simulink subsystem "stack_subsystem_model"  (R2023a)
settings: Solver=VariableStepAuto  StartTime=0.0  StopTime=10.0  RelTol=1e-3
undefined symbols (not defined in the file): constants, coolant_initial_temperature, coolant_num_layers, coolant_num_passes, coolant_w_channels, dewpoint_temperature_degC, env_p, h2_molar_concentration, hydrogen, inlet_flow_lpmin, inlet_pressure_barg, inlet_temperature_degC, oxygen, stack_area, stack_num_cells, stoichiometry
libraries: fl_lib x39, nesl_utility x31
(part 1 of 2)
settings Model: Creator=stefan.notter  LastModifiedBy=adrian.taveras
settings OptimizationCC: ReuseModelBlockBuffer=off

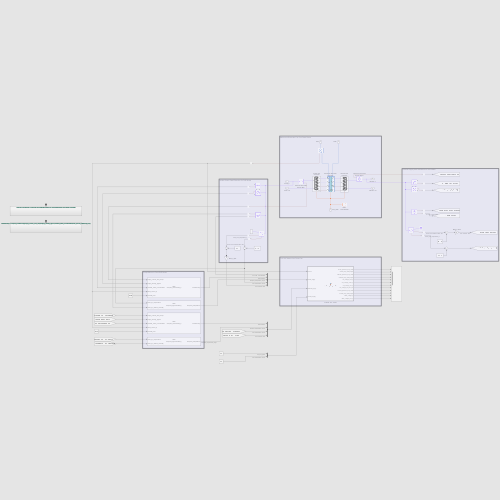
[thumbnail: Simulink's stored preview of the top-level diagram]
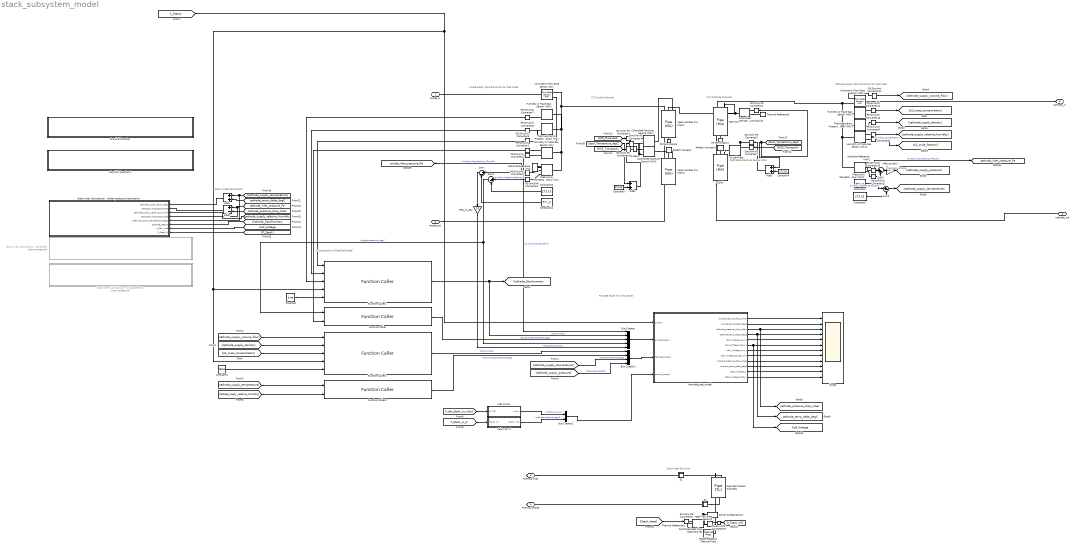
== system stack_subsystem_model ==
  note: Stack-model-Parameters
  note: Computations to Feed DoE Model
  note: Anode Supply Data Extraction for DoE Model
  note: P10 DoE Model from PowerCell
  note: Cathode Supply Data Extraction for DoE Model
  note: FCS Cathode Channels
  note: FCS Anode Channels
  note: Stack Heat Emission
  Absolute Reference (MA) : fl_lib/Moist Air/Elements/Absolute Reference (MA)
  Absolute Reference (MA)1 : fl_lib/Moist Air/Elements/Absolute Reference (MA)
  Add1 : Sum
  Add2 : Sum  Inputs=+-
  Add3 : Sum
  Add4 : Sum
  Bus Creator : BusCreator  Inputs=h2_molar_concentration,stoichiometry,dewpoint_temperature_degC,inlet_temperature_degC,inlet_pressure_barg  OutDataTypeStr=Bus: anode_supply
  Bus Creator1 : BusCreator  Inputs=stoichiometry,dewpoint_temperature_degC,inlet_temperature_degC,inlet_pressure_barg  OutDataTypeStr=Bus: cathode_supply
  Bus Creator2 : BusCreator  Inputs=inlet_flow_lpmin,inlet_temperature_degC  OutDataTypeStr=Bus: coolant_supply
  Cond. : fl_lib/Moist Air/Elements/Pipe (MA)  length=1 m  area=1 m^2  Dh=.1 m  length_add=.1 m  roughness=15e-6 m  Re_lam=2000  Re_tur=4000  shape_factor=64  Nu_lam=3.66  wall_condensation=simscape.enum.onoff.off  RH_ws=1  time_constant=1e-3 s  moisture_trace_gas_source=foundation.enum.moisture_trace_gas_source.controlled  moisture_source_spec=foundation.enum.moisture_source_spec.vapor  moisture_mass_flow=0 kg/s  moisture_temperature_spec=foundation.enum.temperature_spec.atmospheric  moisture_temperature=293.15 K  trace_gas_mass_flow=0 kg/s  trace_gas_temperature_spec=foundation.enum.temperature_spec.atmospheric  trace_gas_temperature=293.15 K  p_I_specify=off  p_I_priority=High  p_I=0.101325 MPa  p_I_nominal_specify=off  p_I_nominal_unit=MPa  p_I_nominal_value=1  T_I_specify=off  T_I_priority=High  T_I=293.15 K  T_I_nominal_specify=off  T_I_nominal_unit=K  T_I_nominal_value=1  RH_I_specify=off  RH_I_priority=High  RH_I=0  RH_I_nominal_specify=off  RH_I_nominal_unit=1  RH_I_nominal_value=1  x_w_I_specify=off  x_w_I_priority=None  x_w_I=0  x_w_I_nominal_specify=off  x_w_I_nominal_unit=1  x_w_I_nominal_value=1  y_w_I_specify=off  y_w_I_priority=None  y_w_I=0  y_w_I_nominal_specify=off  y_w_I_nominal_unit=1  y_w_I_nominal_value=1  HR_I_specify=off  HR_I_priority=None  HR_I=0  HR_I_nominal_specify=off  HR_I_nominal_unit=1  HR_I_nominal_value=1  x_g_I_specify=off  x_g_I_priority=High  x_g_I=0  x_g_I_nominal_specify=off  x_g_I_nominal_unit=1  x_g_I_nominal_value=1  y_g_I_specify=off  y_g_I_priority=None  y_g_I=0  y_g_I_nominal_specify=off  y_g_I_nominal_unit=1  y_g_I_nominal_value=1
      settings: InternalSimscapePortConfiguration="{\"Bottom\":[],\"Left\":[{\"id\":\"A\",\"label\":\"A\",\"type\":\"foundation.moist_air.moist_air\"},{\"id\":\"H\",\"label\":\"H\",\"type\":\"foundation.thermal.thermal\"},{\"id\":\"S\",\"label\":\"S\",\"type\":\"foundation.moist_air.moist_air_source\"}],\"Right\":[{\"id\":\"B\",\"label\":\"B\",\"type\":\"foundation.moist_air.moist_air\"},{\"id\":\"W\",\"label\":\"W\",\"type\":\"output\"},{\"id\":\"F\",\"label\":\"F\",\"type\":\"output\"}],\"Top\":[]}"
  Constant : Constant  Value=true  OutDataTypeStr=boolean
  Constant1 : Constant  Value=false  OutDataTypeStr=boolean
  Constant11 : Constant  Value=env_p
  Constant12 : Constant  Value=273.15
  Constant2 : Constant  Value=env_p
  Constant3 : Constant  Value=273.15
  Constant4 : Constant  Value=273.16
  Constant5 : Constant  Value=273.16
  Controlled Temperature Source : fl_lib/Thermal/Thermal Sources/Controlled Temperature Source
  Controlled Heat Flow Rate Source1 : fl_lib/Thermal/Thermal Sources/Controlled Heat Flow Rate Source
  Controlled Moisture Source (MA)1 : fl_lib/Moist Air/Sources/Moisture & Trace Gas Sources/Controlled Moisture Source (MA)  moisture_source_spec=foundation.enum.moisture_source_spec.vapor  Phi_S_specify=off  Phi_S_priority=None  Phi_S=0 kW  Phi_S_nominal_specify=off  Phi_S_nominal_unit=kW  Phi_S_nominal_value=1  mdot_w_S_specify=off  mdot_w_S_priority=None  mdot_w_S=0 kg/s  mdot_w_S_nominal_specify=off  mdot_w_S_nominal_unit=kg/s  mdot_w_S_nominal_value=1
      settings: InternalSimscapePortConfiguration="{\"Bottom\":[],\"Left\":[{\"id\":\"S\",\"label\":\"S\",\"type\":\"foundation.moist_air.moist_air_source\"}],\"Right\":[{\"id\":\"M\",\"label\":\"M\",\"type\":\"input\"},{\"id\":\"T\",\"label\":\"T\",\"type\":\"input\"}],\"Top\":[]}"
  Controlled Moisture Source (MA)2 : fl_lib/Moist Air/Sources/Moisture & Trace Gas Sources/Controlled Moisture Source (MA)  moisture_source_spec=foundation.enum.moisture_source_spec.vapor  Phi_S_specify=off  Phi_S_priority=None  Phi_S=0 kW  Phi_S_nominal_specify=off  Phi_S_nominal_unit=kW  Phi_S_nominal_value=1  mdot_w_S_specify=off  mdot_w_S_priority=None  mdot_w_S=0 kg/s  mdot_w_S_nominal_specify=off  mdot_w_S_nominal_unit=kg/s  mdot_w_S_nominal_value=1
      settings: InternalSimscapePortConfiguration="{\"Bottom\":[],\"Left\":[{\"id\":\"S\",\"label\":\"S\",\"type\":\"foundation.moist_air.moist_air_source\"}],\"Right\":[{\"id\":\"M\",\"label\":\"M\",\"type\":\"input\"},{\"id\":\"T\",\"label\":\"T\",\"type\":\"input\"}],\"Top\":[]}"
  Fuel Cell Coolant Channels : fl_lib/Thermal Liquid/Elements/Pipe (TL)  length=sqrt(stack_area) * coolant_num_passes cm  area=coolant_w_channels^2 * coolant_num_layers cm^2  Dh=coolant_w_channels cm  length_add=10 cm  roughness=15e-5 m  Re_lam=2000  Re_tur=4000  shape_factor=64  Nu_lam=3.66  dynamic_compressibility=simscape.enum.onoff.on  inertia=simscape.enum.onoff.off  p0=coolant_initial_pressure MPa  T0=coolant_initial_temperature K  mdot0=0 kg/s
  Function Caller : FunctionCaller  FunctionPrototype=dewpoint_temperature = dewpoint_approximation(moist_air_temperature,moist_air_relative_humidity)  InputArgumentSpecifications=<Enter example>  OutputArgumentSpecifications=<Enter example>
  Function Caller1 : FunctionCaller  FunctionPrototype=stoichiometry = compute_stoichiometry(supply_volume_flow_m3ps,supply_density_kgpm3,reactant_mass_concentration,stack_current_A,isanode_bool)  InputArgumentSpecifications=<Enter example>  OutputArgumentSpecifications=<Enter example>
  Function Caller2 : FunctionCaller  FunctionPrototype=stoichiometry = compute_stoichiometry(supply_volume_flow_m3ps,supply_density_kgpm3,reactant_mass_concentration,stack_current_A,isanode_bool)  InputArgumentSpecifications=<Enter example>  OutputArgumentSpecifications=<Enter example>
  Function Caller3 : FunctionCaller  FunctionPrototype=dewpoint_temperature = dewpoint_approximation(moist_air_temperature,moist_air_relative_humidity)  InputArgumentSpecifications=<Enter example>  OutputArgumentSpecifications=<Enter example>
  Heat Flow Rate Sensor1 : fl_lib/Thermal/Thermal Sensors/Heat Flow Rate Sensor
  Humidity & Trace Gas Sensor (MA) : fl_lib/Moist Air/Sensors/Humidity & Trace Gas Sensor (MA)  moisture_on=true  moisture_spec=foundation.enum.moisture_spec.relative_humidity  trace_gas_on=true  trace_gas_spec=foundation.enum.trace_gas_spec.mole_fraction
      settings: InternalSimscapePortConfiguration="{\"Bottom\":[],\"Left\":[{\"id\":\"A\",\"label\":\"A\",\"type\":\"foundation.moist_air.moist_air\"}],\"Right\":[{\"id\":\"W\",\"label\":\"W\",\"type\":\"output\"},{\"id\":\"G\",\"label\":\"G\",\"type\":\"output\"}],\"Top\":[]}"
  Humidity & Trace Gas Sensor (MA)1 : fl_lib/Moist Air/Sensors/Humidity & Trace Gas Sensor (MA)  moisture_on=true  moisture_spec=foundation.enum.moisture_spec.relative_humidity  trace_gas_on=true  trace_gas_spec=foundation.enum.trace_gas_spec.mass_fraction
      settings: InternalSimscapePortConfiguration="{\"Bottom\":[],\"Left\":[{\"id\":\"A\",\"label\":\"A\",\"type\":\"foundation.moist_air.moist_air\"}],\"Right\":[{\"id\":\"W\",\"label\":\"W\",\"type\":\"output\"},{\"id\":\"G\",\"label\":\"G\",\"type\":\"output\"}],\"Top\":[]}"
  Humidity & Trace Gas Sensor (MA)2 : fl_lib/Moist Air/Sensors/Humidity & Trace Gas Sensor (MA)  moisture_on=true  moisture_spec=foundation.enum.moisture_spec.relative_humidity  trace_gas_on=true  trace_gas_spec=foundation.enum.trace_gas_spec.mole_fraction
      settings: InternalSimscapePortConfiguration="{\"Bottom\":[],\"Left\":[{\"id\":\"A\",\"label\":\"A\",\"type\":\"foundation.moist_air.moist_air\"}],\"Right\":[{\"id\":\"W\",\"label\":\"W\",\"type\":\"output\"},{\"id\":\"G\",\"label\":\"G\",\"type\":\"output\"}],\"Top\":[]}"
  Humidity & Trace Gas Sensor (MA)3 : fl_lib/Moist Air/Sensors/Humidity & Trace Gas Sensor (MA)  moisture_on=true  moisture_spec=foundation.enum.moisture_spec.relative_humidity  trace_gas_on=true  trace_gas_spec=foundation.enum.trace_gas_spec.mass_fraction
      settings: InternalSimscapePortConfiguration="{\"Bottom\":[],\"Left\":[{\"id\":\"A\",\"label\":\"A\",\"type\":\"foundation.moist_air.moist_air\"}],\"Right\":[{\"id\":\"W\",\"label\":\"W\",\"type\":\"output\"},{\"id\":\"G\",\"label\":\"G\",\"type\":\"output\"}],\"Top\":[]}"
  Kelvin to °C : Subsystem
  M3s to lpm : Subsystem
  MPa_to_Bar : Gain  Gain=10
  MPa_to_Bar1 : Gain  Gain=10
  PS Gain2 : fl_lib/Physical Signals/Functions/PS Gain  gain=-1
  PS Terminator1 : fl_lib/Physical Signals/Sinks/PS Terminator
  PS Terminator6 : fl_lib/Physical Signals/Sinks/PS Terminator
  PS-Simulink Converter{1..2,4..9,11..14} (12 alike) : nesl_utility/PS-Simulink Converter  PhysicalDomain=network_engine_domain  SubClassName=ps_output  LeftPortType=input  RightPortType=output  PseudoPeriodic=off  Frequencies=[]  VectorFormat=inherit  Unit=inherit  AffineConversion=off
  PS-Simulink Converter10 : nesl_utility/PS-Simulink Converter  PhysicalDomain=network_engine_domain  SubClassName=ps_output  LeftPortType=input  RightPortType=output  PseudoPeriodic=off  Frequencies=[]  VectorFormat=inherit  Unit=MPa  AffineConversion=off
  PS-Simulink Converter16 : nesl_utility/PS-Simulink Converter  PhysicalDomain=network_engine_domain  SubClassName=ps_output  LeftPortType=input  RightPortType=output  PseudoPeriodic=off  Frequencies=[]  VectorFormat=1-D array  Unit=kW  AffineConversion=off
  PS-Simulink Converter3 : nesl_utility/PS-Simulink Converter  PhysicalDomain=network_engine_domain  SubClassName=ps_output  LeftPortType=input  RightPortType=output  PseudoPeriodic=off  Frequencies=[]  VectorFormat=inherit  Unit=MPa  AffineConversion=off
  PS100-P02Stack Thermal Mass : fl_lib/Thermal/Thermal Elements/Thermal Mass  mass_type=foundation.enum.constant_variable.constant  mass=stack_thermal_mass kg  sp_heat=stack_specific_heat J/kg/K  mass_min=1e-6 kg  num_ports=foundation.enum.numPorts2.one  m_specify=off  m_priority=High  m=1 kg  m_nominal_specify=off  m_nominal_unit=kg  m_nominal_value=1  T_specify=on  T_priority=High  T=coolant_initial_temperature K  T_nominal_specify=off  T_nominal_unit=K  T_nominal_value=1  Q_specify=off  Q_priority=None  Q=20e3 W  Q_nominal_specify=off  Q_nominal_unit=W  Q_nominal_value=1
  Perfect Insulator : fl_lib/Thermal/Thermal Elements/Perfect Insulator  T_specify=off  T_priority=None  T=293.15 K  T_nominal_specify=off  T_nominal_unit=K  T_nominal_value=1
  Perfect Insulator1 : fl_lib/Thermal/Thermal Elements/Perfect Insulator  T_specify=off  T_priority=None  T=293.15 K  T_nominal_specify=off  T_nominal_unit=K  T_nominal_value=1
  Pipe (MA) : fl_lib/Moist Air/Elements/Pipe (MA)  length=1 m  area=1 m^2  Dh=.1 m  length_add=.1 m  roughness=15e-6 m  Re_lam=2000  Re_tur=4000  shape_factor=64  Nu_lam=3.66  wall_condensation=simscape.enum.onoff.off  RH_ws=1  time_constant=1e-3 s  moisture_trace_gas_source=foundation.enum.moisture_trace_gas_source.none  moisture_source_spec=foundation.enum.moisture_source_spec.vapor  moisture_mass_flow=0 kg/s  moisture_temperature_spec=foundation.enum.temperature_spec.atmospheric  moisture_temperature=293.15 K  trace_gas_mass_flow=0 kg/s  trace_gas_temperature_spec=foundation.enum.temperature_spec.atmospheric  trace_gas_temperature=293.15 K  p_I_specify=off  p_I_priority=High  p_I=0.101325 MPa  p_I_nominal_specify=off  p_I_nominal_unit=MPa  p_I_nominal_value=1  T_I_specify=off  T_I_priority=High  T_I=293.15 K  T_I_nominal_specify=off  T_I_nominal_unit=K  T_I_nominal_value=1  RH_I_specify=off  RH_I_priority=High  RH_I=0  RH_I_nominal_specify=off  RH_I_nominal_unit=1  RH_I_nominal_value=1  x_w_I_specify=off  x_w_I_priority=None  x_w_I=0  x_w_I_nominal_specify=off  x_w_I_nominal_unit=1  x_w_I_nominal_value=1  y_w_I_specify=off  y_w_I_priority=None  y_w_I=0  y_w_I_nominal_specify=off  y_w_I_nominal_unit=1  y_w_I_nominal_value=1  HR_I_specify=off  HR_I_priority=None  HR_I=0  HR_I_nominal_specify=off  HR_I_nominal_unit=1  HR_I_nominal_value=1  x_g_I_specify=off  x_g_I_priority=High  x_g_I=0  x_g_I_nominal_specify=off  x_g_I_nominal_unit=1  x_g_I_nominal_value=1  y_g_I_specify=off  y_g_I_priority=None  y_g_I=0  y_g_I_nominal_specify=off  y_g_I_nominal_unit=1  y_g_I_nominal_value=1
  Pressure & Temperature Sensor (MA) : fl_lib/Moist Air/Sensors/Pressure & Temperature Sensor (MA)  reference=foundation.enum.MeasurementReference.difference  pressure=true  pressure_spec=foundation.enum.PressureMeasementSpec.Absolute  temperature=true
      settings: InternalSimscapePortConfiguration="{\"Bottom\":[{\"id\":\"T\",\"label\":\"T\",\"type\":\"output\"}],\"Left\":[{\"id\":\"A\",\"label\":\"A\",\"type\":\"foundation.moist_air.moist_air\"}],\"Right\":[{\"id\":\"B\",\"label\":\"B\",\"type\":\"foundation.moist_air.moist_air\"},{\"id\":\"P\",\"label\":\"P\",\"type\":\"output\"}],\"Top\":[]}"
  Pressure & Temperature Sensor (MA)1 : fl_lib/Moist Air/Sensors/Pressure & Temperature Sensor (MA)  reference=foundation.enum.MeasurementReference.difference  pressure=true  pressure_spec=foundation.enum.PressureMeasementSpec.Absolute  temperature=true
      settings: InternalSimscapePortConfiguration="{\"Bottom\":[{\"id\":\"T\",\"label\":\"T\",\"type\":\"output\"}],\"Left\":[{\"id\":\"A\",\"label\":\"A\",\"type\":\"foundation.moist_air.moist_air\"}],\"Right\":[{\"id\":\"B\",\"label\":\"B\",\"type\":\"foundation.moist_air.moist_air\"},{\"id\":\"P\",\"label\":\"P\",\"type\":\"output\"}],\"Top\":[]}"
  S1 : Subsystem
  S2 : Subsystem
  Scope : Scope  NumInputPorts=12
  Simulink Function : Subsystem  TreatAsAtomicUnit=on
  Simulink Function1 : Subsystem  TreatAsAtomicUnit=on
  Simulink-PS Converter : nesl_utility/Simulink-PS Converter  PhysicalDomain=network_engine_domain  SubClassName=ps_input  LeftPortType=input  RightPortType=output  PseudoPeriodic=off  Frequencies=[]  NoiseDistribution=none  NoiseParameters=[]  Unit=1  AffineConversion=off  FilteringAndDerivatives=filter  SimscapeFilterOrder=1  InputFilterTimeConstant=0.001  UdotUserProvided=0
  Simulink-PS Converter1 : nesl_utility/Simulink-PS Converter  PhysicalDomain=network_engine_domain  SubClassName=ps_input  LeftPortType=input  RightPortType=output  PseudoPeriodic=off  Frequencies=[]  NoiseDistribution=none  NoiseParameters=[]  Unit=1  AffineConversion=off  FilteringAndDerivatives=provide  SimscapeFilterOrder=1  InputFilterTimeConstant=0.001  UdotUserProvided=0
  Simulink-PS Converter2 : nesl_utility/Simulink-PS Converter  PhysicalDomain=network_engine_domain  SubClassName=ps_input  LeftPortType=input  RightPortType=output  PseudoPeriodic=off  Frequencies=[]  NoiseDistribution=none  NoiseParameters=[]  Unit=1  AffineConversion=off  FilteringAndDerivatives=filter  SimscapeFilterOrder=1  InputFilterTimeConstant=0.001  UdotUserProvided=0
  Simulink-PS Converter3 : nesl_utility/Simulink-PS Converter  PhysicalDomain=network_engine_domain  SubClassName=ps_input  LeftPortType=input  RightPortType=output  PseudoPeriodic=off  Frequencies=[]  NoiseDistribution=none  NoiseParameters=[]  Unit=1  AffineConversion=off  FilteringAndDerivatives=provide  SimscapeFilterOrder=1  InputFilterTimeConstant=0.001  UdotUserProvided=0
  Simulink-PS Converter4 : nesl_utility/Simulink-PS Converter  PhysicalDomain=network_engine_domain  SubClassName=ps_input  LeftPortType=input  RightPortType=output  PseudoPeriodic=off  Frequencies=[]  NoiseDistribution=none  NoiseParameters=[]  Unit=1  AffineConversion=off  FilteringAndDerivatives=filter  SimscapeFilterOrder=1  InputFilterTimeConstant=0.001  UdotUserProvided=0
  Simulink-PS Converter6 : nesl_utility/Simulink-PS Converter  PhysicalDomain=network_engine_domain  SubClassName=ps_input  LeftPortType=input  RightPortType=output  PseudoPeriodic=off  Frequencies=[]  NoiseDistribution=none  NoiseParameters=[]  Unit=J/s  AffineConversion=off  FilteringAndDerivatives=provide  SimscapeFilterOrder=1  InputFilterTimeConstant=0.001  UdotUserProvided=0
  Simulink-PS Converter7 : nesl_utility/Simulink-PS Converter  PhysicalDomain=network_engine_domain  SubClassName=ps_input  LeftPortType=input  RightPortType=output  PseudoPeriodic=off  Frequencies=[]  NoiseDistribution=none  NoiseParameters=[]  Unit=1  AffineConversion=off  FilteringAndDerivatives=provide  SimscapeFilterOrder=1  InputFilterTimeConstant=0.001  UdotUserProvided=0
  Solver Configuration1 : nesl_utility/Solver Configuration  PhysicalDomain=network_engine_domain  SubClassName=solver  LeftPortType=input  RightPortType=generic  Tones=[]  Harmonics=[]  SimulateNoise=off  Profile=off  UseLocalSampling=off  EnableSwitchedLinearOptims=on  FrequencyDomain=off  UseCCode=off  RelTol=0.001  AbsTol=1e-06  MinStep=1e-09  ToWorkspace=off  RevertToSquareIcSolve=off  NumHomotopyIterations=100  PhasorMode=off  PhasorModeNumHarmonics=1  ConsistencySolver=NEWTON_XTOL_AFTER_FTOL  IndexReductionMethod=DerivativeReplacement  DoDC=off  ResidualTolerance=1e-09  ConsistencyTolSource=GLOBAL  ConsistencyAbsTol=0.001  ConsistencyRelTol=0.001  ConsistencyTolFactor=0.001  UseLocalSolver=on  LocalSolverChoice=NE_BACKWARD_EULER_ADVANCER  ResolveIndetEquations=on  FunctionEvalNumThread=1  LocalSolverSampleTime=0.001  DoFixedCost=on  MaxNonlinIter=3  MaxModeIter=2  ComputeImpulses=off  ImpulseIterations=2  LinearAlgebra=auto  LinearAlgebraNumThread=0  EquationFormulation=NE_TIME_EF  DelaysMemoryBudget=1024  AutomaticFiltering=off  FilteringTimeConstant=0.001  PartitionStorageMethod=AS_NEEDED  PartitionMemoryBudget=1024  PartitionMethod=ROBUST
  Stack Inner Calculations - Simplified : Subsystem  Commented=on
  Stack Inner Calculations - Water production estimation : Subsystem
  Stack Inner Calculations - all parameters : Subsystem  Commented=on
  Sum{,1..3} (4 alike) : Sum  Inputs=|+-
  Thermal Reference1 : fl_lib/Thermal/Thermal Elements/Thermal Reference
  Thermal Reference2 : fl_lib/Thermal/Thermal Elements/Thermal Reference
  Thermodynamic Properties Sensor (MA) : fl_lib/Moist Air/Sensors/Thermodynamic Properties Sensor (MA)  measurement_mass_spec=foundation.enum.measurement_mass_spec.mixture  enthalpy=true  density=true  specific_heat=true  entropy=true
      settings: InternalSimscapePortConfiguration="{\"Bottom\":[{\"id\":\"CP\",\"label\":\"cp\",\"type\":\"output\"},{\"id\":\"S\",\"label\":\"s\",\"type\":\"output\"}],\"Left\":[{\"id\":\"A\",\"label\":\"A\",\"type\":\"foundation.moist_air.moist_air\"}],\"Right\":[{\"id\":\"H\",\"label\":\"h\",\"type\":\"output\"},{\"id\":\"RHO\",\"label\":\"ρ\",\"type\":\"output\"}],\"Top\":[]}"
  Thermodynamic Properties Sensor (MA)1 : fl_lib/Moist Air/Sensors/Thermodynamic Properties Sensor (MA)  measurement_mass_spec=foundation.enum.measurement_mass_spec.mixture  enthalpy=true  density=true  specific_heat=true  entropy=true
      settings: InternalSimscapePortConfiguration="{\"Bottom\":[{\"id\":\"CP\",\"label\":\"cp\",\"type\":\"output\"},{\"id\":\"S\",\"label\":\"s\",\"type\":\"output\"}],\"Left\":[{\"id\":\"A\",\"label\":\"A\",\"type\":\"foundation.moist_air.moist_air\"}],\"Right\":[{\"id\":\"H\",\"label\":\"h\",\"type\":\"output\"},{\"id\":\"RHO\",\"label\":\"ρ\",\"type\":\"output\"}],\"Top\":[]}"
  Vapor and fuel mix (Top)1 : fl_lib/Moist Air/Elements/Pipe (MA)  length=0.25 m  area=pi*0.05^2/4 m^2  Dh=0.05 m  length_add=0.1 m  roughness=15e-6 m  Re_lam=2000  Re_tur=4000  shape_factor=64  Nu_lam=3.66  wall_condensation=simscape.enum.onoff.off  RH_ws=1  time_constant=1e-3 s  moisture_trace_gas_source=foundation.enum.moisture_trace_gas_source.controlled  moisture_source_spec=foundation.enum.moisture_source_spec.vapor  moisture_mass_flow=0 kg/s  moisture_temperature_spec=foundation.enum.temperature_spec.atmospheric  moisture_temperature=293.15 K  trace_gas_mass_flow=0 kg/s  trace_gas_temperature_spec=foundation.enum.temperature_spec.atmospheric  trace_gas_temperature=293.15 K  p_I_specify=on  p_I_priority=High  p_I=env_p MPa  p_I_nominal_specify=off  p_I_nominal_unit=MPa  p_I_nominal_value=1  T_I_specify=on  T_I_priority=High  T_I=env_T degC  T_I_nominal_specify=off  T_I_nominal_unit=K  T_I_nominal_value=1  RH_I_specify=off  RH_I_priority=High  RH_I=0  RH_I_nominal_specify=off  RH_I_nominal_unit=1  RH_I_nominal_value=1  x_w_I_specify=off  x_w_I_priority=None  x_w_I=0  x_w_I_nominal_specify=off  x_w_I_nominal_unit=1  x_w_I_nominal_value=1  y_w_I_specify=off  y_w_I_priority=None  y_w_I=0  y_w_I_nominal_specify=off  y_w_I_nominal_unit=1  y_w_I_nominal_value=1  HR_I_specify=off  HR_I_priority=None  HR_I=0  HR_I_nominal_specify=off  HR_I_nominal_unit=1  HR_I_nominal_value=1  x_g_I_specify=on  x_g_I_priority=None  x_g_I=0  x_g_I_nominal_specify=off  x_g_I_nominal_unit=1  x_g_I_nominal_value=1  y_g_I_specify=on  y_g_I_priority=High  y_g_I=tank_yH2  y_g_I_nominal_specify=off  y_g_I_nominal_unit=1  y_g_I_nominal_value=1
      settings: InternalSimscapePortConfiguration="{\"Bottom\":[],\"Left\":[{\"id\":\"A\",\"label\":\"A\",\"type\":\"foundation.moist_air.moist_air\"},{\"id\":\"H\",\"label\":\"H\",\"type\":\"foundation.thermal.thermal\"},{\"id\":\"S\",\"label\":\"S\",\"type\":\"foundation.moist_air.moist_air_source\"}],\"Right\":[{\"id\":\"B\",\"label\":\"B\",\"type\":\"foundation.moist_air.moist_air\"},{\"id\":\"W\",\"label\":\"W\",\"type\":\"output\"},{\"id\":\"F\",\"label\":\"F\",\"type\":\"output\"}],\"Top\":[]}"
  Vapor and fuel mix (Top)2 : fl_lib/Moist Air/Elements/Pipe (MA)  length=0.25 m  area=pi*0.05^2/4 m^2  Dh=0.05 m  length_add=0.1 m  roughness=15e-6 m  Re_lam=2000  Re_tur=4000  shape_factor=64  Nu_lam=3.66  wall_condensation=simscape.enum.onoff.off  RH_ws=1  time_constant=1e-3 s  moisture_trace_gas_source=foundation.enum.moisture_trace_gas_source.controlled  moisture_source_spec=foundation.enum.moisture_source_spec.vapor  moisture_mass_flow=0 kg/s  moisture_temperature_spec=foundation.enum.temperature_spec.atmospheric  moisture_temperature=293.15 K  trace_gas_mass_flow=0 kg/s  trace_gas_temperature_spec=foundation.enum.temperature_spec.atmospheric  trace_gas_temperature=293.15 K  p_I_specify=on  p_I_priority=High  p_I=env_p MPa  p_I_nominal_specify=off  p_I_nominal_unit=MPa  p_I_nominal_value=1  T_I_specify=on  T_I_priority=High  T_I=env_T degC  T_I_nominal_specify=off  T_I_nominal_unit=K  T_I_nominal_value=1  RH_I_specify=off  RH_I_priority=High  RH_I=0  RH_I_nominal_specify=off  RH_I_nominal_unit=1  RH_I_nominal_value=1  x_w_I_specify=off  x_w_I_priority=None  x_w_I=0  x_w_I_nominal_specify=off  x_w_I_nominal_unit=1  x_w_I_nominal_value=1  y_w_I_specify=off  y_w_I_priority=None  y_w_I=0  y_w_I_nominal_specify=off  y_w_I_nominal_unit=1  y_w_I_nominal_value=1  HR_I_specify=off  HR_I_priority=None  HR_I=0  HR_I_nominal_specify=off  HR_I_nominal_unit=1  HR_I_nominal_value=1  x_g_I_specify=on  x_g_I_priority=None  x_g_I=0  x_g_I_nominal_specify=off  x_g_I_nominal_unit=1  x_g_I_nominal_value=1  y_g_I_specify=on  y_g_I_priority=High  y_g_I=tank_yH2  y_g_I_nominal_specify=off  y_g_I_nominal_unit=1  y_g_I_nominal_value=1
      settings: InternalSimscapePortConfiguration="{\"Bottom\":[],\"Left\":[{\"id\":\"A\",\"label\":\"A\",\"type\":\"foundation.moist_air.moist_air\"},{\"id\":\"H\",\"label\":\"H\",\"type\":\"foundation.thermal.thermal\"},{\"id\":\"S\",\"label\":\"S\",\"type\":\"foundation.moist_air.moist_air_source\"}],\"Right\":[{\"id\":\"B\",\"label\":\"B\",\"type\":\"foundation.moist_air.moist_air\"},{\"id\":\"W\",\"label\":\"W\",\"type\":\"output\"},{\"id\":\"F\",\"label\":\"F\",\"type\":\"output\"}],\"Top\":[]}"
  Volumetric Flow Rate Sensor (MA) : fl_lib/Moist Air/Sensors/Flow Rate Sensor (MA)  mass_flow_measure=false  volumetric_flow_measure=true  volumetric_flow_conditions=foundation.enum.volumetric_flow_conditions.actual  p_std=0.101325 MPa  T_std=20 degC  RH_std=0.65  energy_flow_measure=false  vapor_flow_measure=false  gas_flow_measure=false
      settings: InternalSimscapePortConfiguration="{\"Bottom\":[],\"Left\":[{\"id\":\"A\",\"label\":\"A\",\"type\":\"foundation.moist_air.moist_air\"}],\"Right\":[{\"id\":\"B\",\"label\":\"B\",\"type\":\"foundation.moist_air.moist_air\"},{\"id\":\"V\",\"label\":\"V\",\"type\":\"output\"}],\"Top\":[]}"
  Volumetric Flow Rate Sensor (MA)1 : fl_lib/Moist Air/Sensors/Flow Rate Sensor (MA)  mass_flow_measure=false  volumetric_flow_measure=true  volumetric_flow_conditions=foundation.enum.volumetric_flow_conditions.actual  p_std=0.101325 MPa  T_std=20 degC  RH_std=0.65  energy_flow_measure=false  vapor_flow_measure=false  gas_flow_measure=false
      settings: InternalSimscapePortConfiguration="{\"Bottom\":[],\"Left\":[{\"id\":\"A\",\"label\":\"A\",\"type\":\"foundation.moist_air.moist_air\"}],\"Right\":[{\"id\":\"B\",\"label\":\"B\",\"type\":\"foundation.moist_air.moist_air\"},{\"id\":\"V\",\"label\":\"V\",\"type\":\"output\"}],\"Top\":[]}"
  W_add Rate : fl_lib/Moist Air/Sources/Moisture & Trace Gas Sources/Controlled Moisture Source (MA)  moisture_source_spec=foundation.enum.moisture_source_spec.liquid  Phi_S_specify=off  Phi_S_priority=None  Phi_S=0 kW  Phi_S_nominal_specify=off  Phi_S_nominal_unit=kW  Phi_S_nominal_value=1  mdot_w_S_specify=off  mdot_w_S_priority=None  mdot_w_S=0 kg/s  mdot_w_S_nominal_specify=off  mdot_w_S_nominal_unit=kg/s  mdot_w_S_nominal_value=1
      settings: InternalSimscapePortConfiguration="{\"Bottom\":[],\"Left\":[{\"id\":\"S\",\"label\":\"S\",\"type\":\"foundation.moist_air.moist_air_source\"}],\"Right\":[{\"id\":\"M\",\"label\":\"M\",\"type\":\"input\"},{\"id\":\"T\",\"label\":\"T\",\"type\":\"input\"}],\"Top\":[]}"
  evaluate_doe_model : MATLAB Function  TreatAsAtomicUnit=on
  anode_in : PMIOPort  Side=Left
  anode_out : PMIOPort  Port=2  Side=Left
  cathode_in : PMIOPort  Port=3  Side=Right
  cathode_out : PMIOPort  Port=4  Side=Right
  Thermal Inlet : PMIOPort  Port=5  Side=Left
  Thermal Outlet : PMIOPort  Port=6  Side=Left
  tag scope: Cathode_Stochiometry=global, Cell_Voltage=global, Q_Stack_kW=global, anode_inlet_pressure_Pa=global, cathode_inlet_pressure_Pa=global, cathode_pressure_drop_mbar=global, cathode_temp_delta_degC=global
  wires:
  evaluate_doe_model/8(cell_voltage_std_dev_mV) -> Scope/8
  evaluate_doe_model/1(anode_pressure_drop_mbar) -> Scope/1
  evaluate_doe_model/2(anode_temp_delta_degC) -> Scope/2
  evaluate_doe_model/3(cathode_pressure_drop_mbar) -> Scope/3, [cathode_pressure_drop_mbar]
  evaluate_doe_model/4(cathode_temp_delta_degC) -> Scope/4, [cathode_temp_delta_degC]
  evaluate_doe_model/5(cell_voltage_max_V) -> Scope/5
  evaluate_doe_model/6(cell_voltage_mean_V) -> Scope/6, [Cell_Voltage]
  evaluate_doe_model/7(cell_voltage_min_V) -> Scope/7
  evaluate_doe_model/9(coolant_pressure_drop_mbar) -> Scope/9
  evaluate_doe_model/10(coolant_temp_delta_degC) -> Scope/10
  evaluate_doe_model/11(stack_voltage_V) -> Scope/11
  evaluate_doe_model/12(stack_voltage_loss_V) -> Scope/12
  Bus Creator/1 -> evaluate_doe_model/2(anode_supply)
  Function Caller1/1 -> [Cathode_Stochiometry], Bus Creator/2  "stoichiometry"
  Function Caller/1 -> Bus Creator/3  "dewpoint_temperature_degC"
  [cathode_supply_pressure] -> Bus Creator1/4  "inlet_pressure_barg"
  [cathode_supply_temperature] -> Bus Creator1/3  "inlet_temperature_degC"
  Function Caller3/1 -> Bus Creator1/2  "dewpoint_temperature_degC"
  Function Caller2/1 -> Bus Creator1/1  "stoichiometry"
  Bus Creator1/1 -> evaluate_doe_model/3(cathode_supply)
  Bus Creator2/1 -> evaluate_doe_model/4(coolant_supply)
  M3s to lpm/1(L/min) -> Bus Creator2/1  "inlet_flow_lpmin"
  Kelvin to °C/1(Temp. (°C)) -> Bus Creator2/2  "inlet_temperature_degC"
  [i_Stack] -> evaluate_doe_model/1(current), Function Caller1/4, Function Caller2/4
  PS-Simulink Converter3/1 -> Sum/1, [anode_inlet_pressure_Pa]  "anode_inlet_pressure_MPa_abs"
  Constant11/1 -> Sum/2
  Sum/1 -> MPa_to_Bar/1
  PS-Simulink Converter4/1 -> Sum1/1  "anode_inlet_temperature_K"
  Constant12/1 -> Sum1/2
  PS-Simulink Converter2/1 -> Bus Creator/1  "h2_molar_concentration"
  MPa_to_Bar/1 -> Bus Creator/5  "inlet_pressure_barg"
  Sum1/1 -> Function Caller/1, Bus Creator/4  "inlet_temperature_degC"
  PS-Simulink Converter1/1 -> Function Caller/2
  PS-Simulink Converter5/1 -> Function Caller1/1
  Constant/1 -> Function Caller1/5
  PS-Simulink Converter6/1 -> Function Caller1/2
  PS-Simulink Converter7/1 -> Function Caller1/3
  Constant1/1 -> Function Caller2/5
  PS-Simulink Converter10/1 -> Sum2/1, [cathode_inlet_pressure_Pa]  "anode_inlet_pressure_MPa_abs"
  Constant2/1 -> Sum2/2
  PS-Simulink Converter11/1 -> Sum3/1  "anode_inlet_temperature_K"
  Constant3/1 -> Sum3/2
  PS-Simulink Converter14/1 -> [o2_mass_concentration]
  PS-Simulink Converter13/1 -> [cathode_supply_density]
  PS-Simulink Converter8/1 -> [cathode_supply_relative_humidity]
  PS-Simulink Converter9/1 -> [o2_mole_fraction]  "h2_molar_concentration"
  PS-Simulink Converter12/1 -> [cathode_supply_volume_flow]
  [o2_mass_concentration] -> Function Caller2/3
  [cathode_supply_density] -> Function Caller2/2
  [cathode_supply_volume_flow] -> Function Caller2/1
  Sum2/1 -> MPa_to_Bar1/1
  MPa_to_Bar1/1 -> [cathode_supply_pressure]  "inlet_pressure_barg"
  Sum3/1 -> [cathode_supply_temperature]
  [cathode_supply_temperature] -> Function Caller3/1
  [cathode_supply_relative_humidity] -> Function Caller3/2
  [Stack_Heat] -> Simulink-PS Converter6/1
  PS-Simulink Converter16/1 -> [Q_Stack_kW]
  [T_Stack_in_K] -> Kelvin to °C/1(Temp. (K))
  [vdot_Stack_in_m3s] -> M3s to lpm/1(M^3/S)
  [H2O_Produced] -> Simulink-PS Converter1/1
  [H20_Transport] -> Simulink-PS Converter3/1
  [H20_Transport] -> Simulink-PS Converter7/1
  Add1/1 -> Stack Inner Calculations - Water production estimation/1(cathode_supply_temp_degC)
  Add2/1 -> Stack Inner Calculations - Water production estimation/2(cathode_inlet_pressure_Pa)
  [cathode_supply_temperature] -> Stack Inner Calculations - Water production estimation/5(Cathode_supply_temperature_degC), Add1/1
  [cathode_inlet_pressure_Pa] -> Stack Inner Calculations - Water production estimation/4(Cathode_inlet_pressure_Pa), Add2/1
  [cathode_supply_relative_humidity] -> Stack Inner Calculations - Water production estimation/3(cathode_supply_relative_humidity)
  [Cathode_Stochiometry] -> Stack Inner Calculations - Water production estimation/6(Cathode_OER_%)
  [cathode_temp_delta_degC] -> Add1/2
  [cathode_pressure_drop_mbar] -> Add2/2
  [Cell_Voltage] -> Stack Inner Calculations - Water production estimation/7(V_Cell_volts)
  [P_Stack] -> Stack Inner Calculations - Water production estimation/8(P_Stack_W)
  [Stack_Temperature_degC] -> Add3/1, Simulink-PS Converter4/1
  Constant4/1 -> Add3/2
  Add3/1 -> Simulink-PS Converter2/1
  [Stack_Temperature_degC] -> Add4/1
  Constant5/1 -> Add4/2
  Add4/1 -> Simulink-PS Converter/1
  connections:
  Fuel Cell Coolant Channels/LConn2 -- Heat Flow Rate Sensor1/RConn2 -- PS100-P02Stack Thermal Mass/LConn1
  Solver Configuration1/RConn1 -- Controlled Heat Flow Rate Source1/LConn1 -- Heat Flow Rate Sensor1/LConn1
  Pressure & Temperature Sensor (MA)/LConn1 -- Volumetric Flow Rate Sensor (MA)/RConn1 -- Vapor and fuel mix (Top)1/LConn1 -- Humidity & Trace Gas Sensor (MA)1/LConn1 -- Thermodynamic Properties Sensor (MA)/LConn1 -- Humidity & Trace Gas Sensor (MA)/LConn1
  Pressure & Temperature Sensor (MA)1/LConn1 -- Volumetric Flow Rate Sensor (MA)1/RConn1 -- Pipe (MA)/LConn1 -- Humidity & Trace Gas Sensor (MA)3/LConn1 -- Thermodynamic Properties Sensor (MA)1/LConn1 -- Humidity & Trace Gas Sensor (MA)2/LConn1
  Controlled Moisture Source (MA)2/RConn2 -- Controlled Moisture Source (MA)1/RConn2 -- Simulink-PS Converter/RConn1
  W_add Rate/RConn2 -- Simulink-PS Converter2/RConn1
  Controlled Temperature Source/LConn1 -- Vapor and fuel mix (Top)1/LConn2 -- Pipe (MA)/LConn2
  Volumetric Flow Rate Sensor (MA)1/LConn1 -- cathode_in/RConn1
  Humidity & Trace Gas Sensor (MA)/RConn2 -- PS-Simulink Converter2/LConn1
  PS-Simulink Converter3/LConn1 -- Pressure & Temperature Sensor (MA)/RConn2
  PS-Simulink Converter4/LConn1 -- Pressure & Temperature Sensor (MA)/RConn3
  Absolute Reference (MA)/LConn1 -- Pressure & Temperature Sensor (MA)/RConn1
  PS-Simulink Converter1/LConn1 -- Humidity & Trace Gas Sensor (MA)/RConn1
  Volumetric Flow Rate Sensor (MA)/RConn2 -- PS-Simulink Converter5/LConn1
  Thermodynamic Properties Sensor (MA)/RConn2 -- PS-Simulink Converter6/LConn1
  PS-Simulink Converter7/LConn1 -- Humidity & Trace Gas Sensor (MA)1/RConn2
  PS-Simulink Converter14/LConn1 -- Humidity & Trace Gas Sensor (MA)3/RConn2
  PS-Simulink Converter8/LConn1 -- Humidity & Trace Gas Sensor (MA)2/RConn1
  PS-Simulink Converter10/LConn1 -- Pressure & Temperature Sensor (MA)1/RConn2
  Absolute Reference (MA)1/LConn1 -- Pressure & Temperature Sensor (MA)1/RConn1
  Humidity & Trace Gas Sensor (MA)2/RConn2 -- PS-Simulink Converter9/LConn1
  Thermodynamic Properties Sensor (MA)1/RConn2 -- PS-Simulink Converter13/LConn1
  Volumetric Flow Rate Sensor (MA)1/RConn2 -- PS-Simulink Converter12/LConn1
  Pressure & Temperature Sensor (MA)1/RConn3 -- PS-Simulink Converter11/LConn1
  Cond./LConn2 -- Perfect Insulator1/LConn1
  Pipe (MA)/RConn1 -- Cond./LConn1
  W_add Rate/LConn1 -- Cond./LConn3
  Vapor and fuel mix (Top)1/RConn2 -- PS Terminator6/LConn1
  anode_out/RConn1 -- Vapor and fuel mix (Top)2/RConn1
  Cond./RConn1 -- cathode_out/RConn1
  S2/LConn1 -- Fuel Cell Coolant Channels/RConn1
  S1/RConn1 -- Fuel Cell Coolant Channels/LConn1
  Thermal Inlet/RConn1 -- S1/LConn1
  Thermal Reference1/LConn1 -- Controlled Heat Flow Rate Source1/RConn2
  Simulink-PS Converter6/RConn1 -- Controlled Heat Flow Rate Source1/RConn1
  Heat Flow Rate Sensor1/RConn1 -- PS-Simulink Converter16/LConn1
  S2/RConn1 -- Thermal Outlet/RConn1
  anode_in/RConn1 -- Volumetric Flow Rate Sensor (MA)/LConn1
  Vapor and fuel mix (Top)2/LConn1 -- Vapor and fuel mix (Top)1/RConn1
  Vapor and fuel mix (Top)1/LConn3 -- Controlled Moisture Source (MA)1/LConn1
  Controlled Moisture Source (MA)1/RConn1 -- Simulink-PS Converter1/RConn1
  PS Gain2/RConn1 -- Controlled Moisture Source (MA)2/RConn1
  Simulink-PS Converter3/RConn1 -- PS Gain2/LConn1
  Controlled Moisture Source (MA)2/LConn1 -- Vapor and fuel mix (Top)2/LConn3
  PS Terminator1/LConn1 -- Pipe (MA)/RConn2
  Simulink-PS Converter7/RConn1 -- W_add Rate/RConn1
  Vapor and fuel mix (Top)2/LConn2 -- Perfect Insulator/LConn1
  Controlled Temperature Source/RConn2 -- Thermal Reference2/LConn1
  Simulink-PS Converter4/RConn1 -- Controlled Temperature Source/RConn1

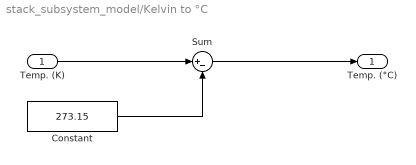
== system stack_subsystem_model/Kelvin to °C ==
  Temp. (K) : Inport
  Constant : Constant  Value=273.15
  Sum : Sum  Inputs=|+-
  Temp. (°C) : Outport
  wires:
  Temp. (K)/1 -> Sum/1
  Sum/1 -> Temp. (°C)/1
  Constant/1 -> Sum/2

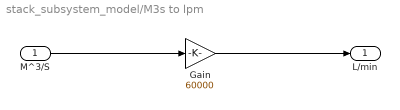
== system stack_subsystem_model/M3s to lpm ==
  M^3/S : Inport
  Gain : Gain  Gain=60000
  L/min : Outport
  wires:
  Gain/1 -> L/min/1
  M^3/S/1 -> Gain/1

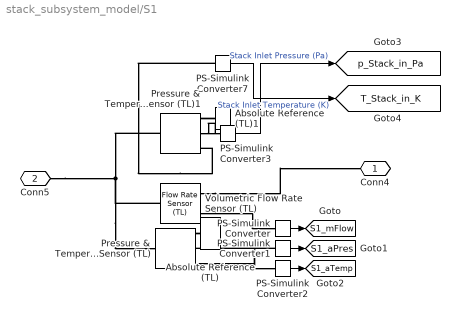
== system stack_subsystem_model/S1 ==
  Absolute Reference (TL) : fl_lib/Thermal Liquid/Elements/Absolute Reference (TL)
  Absolute Reference (TL)1 : fl_lib/Thermal Liquid/Elements/Absolute Reference (TL)
  PS-Simulink Converter{,1..3,7} (5 alike) : nesl_utility/PS-Simulink Converter  PhysicalDomain=network_engine_domain  SubClassName=ps_output  LeftPortType=input  RightPortType=output  PseudoPeriodic=off  Frequencies=[]  VectorFormat=inherit  Unit=inherit  AffineConversion=off
  Pressure & Temperature Sensor (TL) : fl_lib/Thermal Liquid/Sensors/Pressure & Temperature Sensor (TL)  reference=foundation.enum.MeasurementReference.difference  pressure=true  pressure_spec=foundation.enum.PressureMeasementSpec.Absolute  temperature=true
      settings: InternalSimscapePortConfiguration="{\"Bottom\":[{\"id\":\"T\",\"label\":\"T\",\"type\":\"output\"}],\"Left\":[{\"id\":\"A\",\"label\":\"A\",\"type\":\"foundation.thermal_liquid.thermal_liquid\"}],\"Right\":[{\"id\":\"B\",\"label\":\"B\",\"type\":\"foundation.thermal_liquid.thermal_liquid\"},{\"id\":\"P\",\"label\":\"P\",\"type\":\"output\"}],\"Top\":[]}"
  Pressure & Temperature Sensor (TL)1 : fl_lib/Thermal Liquid/Sensors/Pressure & Temperature Sensor (TL)  reference=foundation.enum.MeasurementReference.difference  pressure=true  pressure_spec=foundation.enum.PressureMeasementSpec.Absolute  temperature=true
      settings: InternalSimscapePortConfiguration="{\"Bottom\":[{\"id\":\"T\",\"label\":\"T\",\"type\":\"output\"}],\"Left\":[{\"id\":\"A\",\"label\":\"A\",\"type\":\"foundation.thermal_liquid.thermal_liquid\"}],\"Right\":[{\"id\":\"B\",\"label\":\"B\",\"type\":\"foundation.thermal_liquid.thermal_liquid\"},{\"id\":\"P\",\"label\":\"P\",\"type\":\"output\"}],\"Top\":[]}"
  Volumetric Flow Rate Sensor (TL) : fl_lib/Thermal Liquid/Sensors/Flow Rate Sensor (TL)  mass_flow_measure=false  volumetric_flow_measure=true  energy_flow_measure=false
      settings: InternalSimscapePortConfiguration="{\"Bottom\":[],\"Left\":[{\"id\":\"A\",\"label\":\"A\",\"type\":\"foundation.thermal_liquid.thermal_liquid\"}],\"Right\":[{\"id\":\"B\",\"label\":\"B\",\"type\":\"foundation.thermal_liquid.thermal_liquid\"},{\"id\":\"V\",\"label\":\"V\",\"type\":\"output\"}],\"Top\":[]}"
  Conn4 : PMIOPort  Side=Right
  Conn5 : PMIOPort  Port=2  Side=Left
  tag scope: S1_aPres=global, S1_aTemp=global, S1_mFlow=global, T_Stack_in_K=global, p_Stack_in_Pa=global
  wires:
  PS-Simulink Converter1/1 -> [S1_aPres]
  PS-Simulink Converter2/1 -> [S1_aTemp]
  PS-Simulink Converter/1 -> [S1_mFlow]
  PS-Simulink Converter3/1 -> [p_Stack_in_Pa]  "Stack Inlet Pressure (Pa)"
  PS-Simulink Converter7/1 -> [T_Stack_in_K]  "Stack Inlet Temperature (K)"
  connections:
  Volumetric Flow Rate Sensor (TL)/RConn2 -- PS-Simulink Converter/LConn1
  Volumetric Flow Rate Sensor (TL)/RConn1 -- Conn4/RConn1
  Pressure & Temperature Sensor (TL)/RConn3 -- PS-Simulink Converter2/LConn1
  Pressure & Temperature Sensor (TL)/LConn1 -- Volumetric Flow Rate Sensor (TL)/LConn1 -- Conn5/RConn1 -- Pressure & Temperature Sensor (TL)1/LConn1
  PS-Simulink Converter1/LConn1 -- Pressure & Temperature Sensor (TL)/RConn2
  Absolute Reference (TL)/LConn1 -- Pressure & Temperature Sensor (TL)/RConn1
  PS-Simulink Converter7/LConn1 -- Pressure & Temperature Sensor (TL)1/RConn3
  Pressure & Temperature Sensor (TL)1/RConn2 -- PS-Simulink Converter3/LConn1
  Absolute Reference (TL)1/LConn1 -- Pressure & Temperature Sensor (TL)1/RConn1

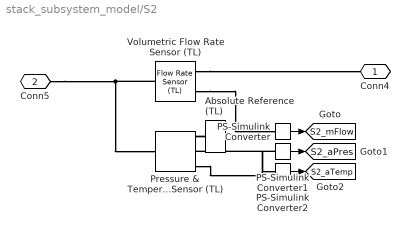
== system stack_subsystem_model/S2 ==
  Absolute Reference (TL) : fl_lib/Thermal Liquid/Elements/Absolute Reference (TL)
  PS-Simulink Converter : nesl_utility/PS-Simulink Converter  PhysicalDomain=network_engine_domain  SubClassName=ps_output  LeftPortType=input  RightPortType=output  PseudoPeriodic=off  Frequencies=[]  VectorFormat=inherit  Unit=inherit  AffineConversion=off
  PS-Simulink Converter1 : nesl_utility/PS-Simulink Converter  PhysicalDomain=network_engine_domain  SubClassName=ps_output  LeftPortType=input  RightPortType=output  PseudoPeriodic=off  Frequencies=[]  VectorFormat=inherit  Unit=inherit  AffineConversion=off
  PS-Simulink Converter2 : nesl_utility/PS-Simulink Converter  PhysicalDomain=network_engine_domain  SubClassName=ps_output  LeftPortType=input  RightPortType=output  PseudoPeriodic=off  Frequencies=[]  VectorFormat=inherit  Unit=inherit  AffineConversion=off
  Pressure & Temperature Sensor (TL) : fl_lib/Thermal Liquid/Sensors/Pressure & Temperature Sensor (TL)  reference=foundation.enum.MeasurementReference.difference  pressure=true  pressure_spec=foundation.enum.PressureMeasementSpec.Absolute  temperature=true
      settings: InternalSimscapePortConfiguration="{\"Bottom\":[{\"id\":\"T\",\"label\":\"T\",\"type\":\"output\"}],\"Left\":[{\"id\":\"A\",\"label\":\"A\",\"type\":\"foundation.thermal_liquid.thermal_liquid\"}],\"Right\":[{\"id\":\"B\",\"label\":\"B\",\"type\":\"foundation.thermal_liquid.thermal_liquid\"},{\"id\":\"P\",\"label\":\"P\",\"type\":\"output\"}],\"Top\":[]}"
  Volumetric Flow Rate Sensor (TL) : fl_lib/Thermal Liquid/Sensors/Flow Rate Sensor (TL)  mass_flow_measure=false  volumetric_flow_measure=true  energy_flow_measure=false
      settings: InternalSimscapePortConfiguration="{\"Bottom\":[],\"Left\":[{\"id\":\"A\",\"label\":\"A\",\"type\":\"foundation.thermal_liquid.thermal_liquid\"}],\"Right\":[{\"id\":\"B\",\"label\":\"B\",\"type\":\"foundation.thermal_liquid.thermal_liquid\"},{\"id\":\"V\",\"label\":\"V\",\"type\":\"output\"}],\"Top\":[]}"
  Conn4 : PMIOPort  Side=Right
  Conn5 : PMIOPort  Port=2  Side=Left
  tag scope: S2_aPres=global, S2_aTemp=global, S2_mFlow=global
  wires:
  PS-Simulink Converter/1 -> [S2_mFlow]
  PS-Simulink Converter2/1 -> [S2_aTemp]
  PS-Simulink Converter1/1 -> [S2_aPres]
  connections:
  Conn5/RConn1 -- Volumetric Flow Rate Sensor (TL)/LConn1 -- Pressure & Temperature Sensor (TL)/LConn1
  Pressure & Temperature Sensor (TL)/RConn3 -- PS-Simulink Converter2/LConn1
  PS-Simulink Converter1/LConn1 -- Pressure & Temperature Sensor (TL)/RConn2
  Volumetric Flow Rate Sensor (TL)/RConn1 -- Conn4/RConn1
  Volumetric Flow Rate Sensor (TL)/RConn2 -- PS-Simulink Converter/LConn1
  Absolute Reference (TL)/LConn1 -- Pressure & Temperature Sensor (TL)/RConn1

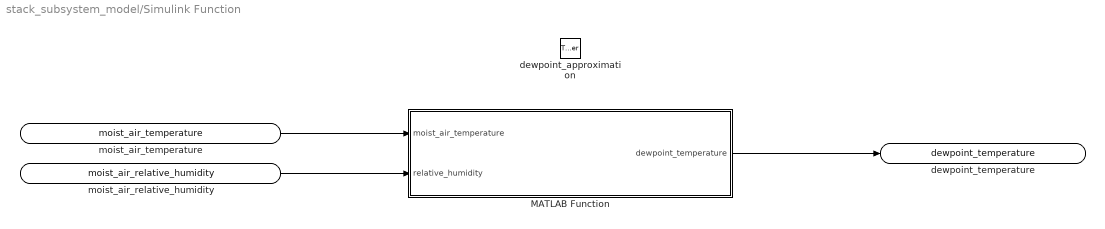
== system stack_subsystem_model/Simulink Function ==
  dewpoint_approximation : TriggerPort  TriggerType=function-call  IsSimulinkFunction=on  FunctionName=dewpoint_approximation  FunctionVisibility=scoped  VariantControl=(inherit)
  MATLAB Function : MATLAB Function  TreatAsAtomicUnit=on
  moist_air_temperature : ArgIn  DisableCoverage=on  ArgumentName=moist_air_temperature
  moist_air_relative_humidity : ArgIn  DisableCoverage=on  Port=2  ArgumentName=moist_air_relative_humidity
  dewpoint_temperature : ArgOut  DisableCoverage=on  ArgumentName=dewpoint_temperature
  wires:
  moist_air_relative_humidity/1 -> MATLAB Function/2(relative_humidity)
  moist_air_temperature/1 -> MATLAB Function/1(moist_air_temperature)
  MATLAB Function/1(dewpoint_temperature) -> dewpoint_temperature/1

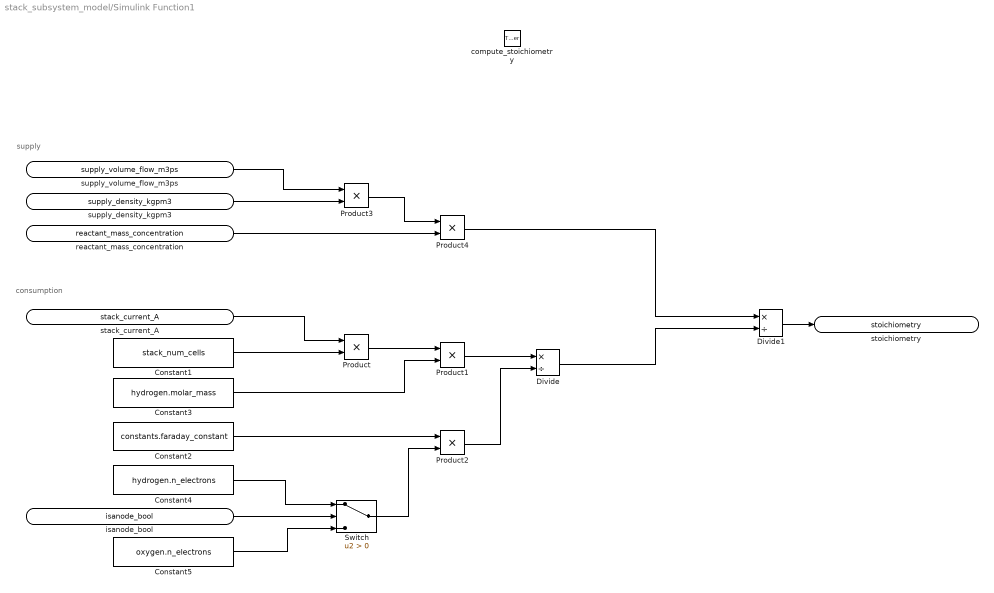
== system stack_subsystem_model/Simulink Function1 ==
  note: consumption
  note: supply
  compute_stoichiometry : TriggerPort  TriggerType=function-call  IsSimulinkFunction=on  FunctionName=compute_stoichiometry  FunctionVisibility=scoped  VariantControl=(inherit)
  Constant1 : Constant  Value=stack_num_cells
  Constant2 : Constant  Value=constants.faraday_constant
  Constant3 : Constant  Value=hydrogen.molar_mass
  Constant4 : Constant  Value=hydrogen.n_electrons
  Constant5 : Constant  Value=oxygen.n_electrons
  Divide : Product  Inputs=*/  RndMeth=Zero  SaturateOnIntegerOverflow=on
  Divide1 : Product  Inputs=*/  RndMeth=Zero  SaturateOnIntegerOverflow=on
  Product{,1..4} (5 alike) : Product
  Switch : Switch  Criteria=u2 > Threshold  SaturateOnIntegerOverflow=off  InputSameDT=off
  supply_volume_flow_m3ps : ArgIn  DisableCoverage=on  ArgumentName=supply_volume_flow_m3ps
  supply_density_kgpm3 : ArgIn  DisableCoverage=on  Port=2  ArgumentName=supply_density_kgpm3
  reactant_mass_concentration : ArgIn  DisableCoverage=on  Port=3  ArgumentName=reactant_mass_concentration
  stack_current_A : ArgIn  DisableCoverage=on  Port=4  ArgumentName=stack_current_A
  isanode_bool : ArgIn  DisableCoverage=on  Port=5  OutDataTypeStr=boolean  ArgumentName=isanode_bool
  stoichiometry : ArgOut  DisableCoverage=on  ArgumentName=stoichiometry
  wires:
  Divide/1 -> Divide1/2
  Product4/1 -> Divide1/1
  Product3/1 -> Product4/1
  reactant_mass_concentration/1 -> Product4/2
  supply_density_kgpm3/1 -> Product3/2
  supply_volume_flow_m3ps/1 -> Product3/1
  Product2/1 -> Divide/2
  Switch/1 -> Product2/2
  Constant5/1 -> Switch/3
  Constant4/1 -> Switch/1
  isanode_bool/1 -> Switch/2
  Constant3/1 -> Product1/2
  Constant2/1 -> Product2/1
  Product1/1 -> Divide/1
  Constant1/1 -> Product/2
  Product/1 -> Product1/1
  Divide1/1 -> stoichiometry/1
  stack_current_A/1 -> Product/1

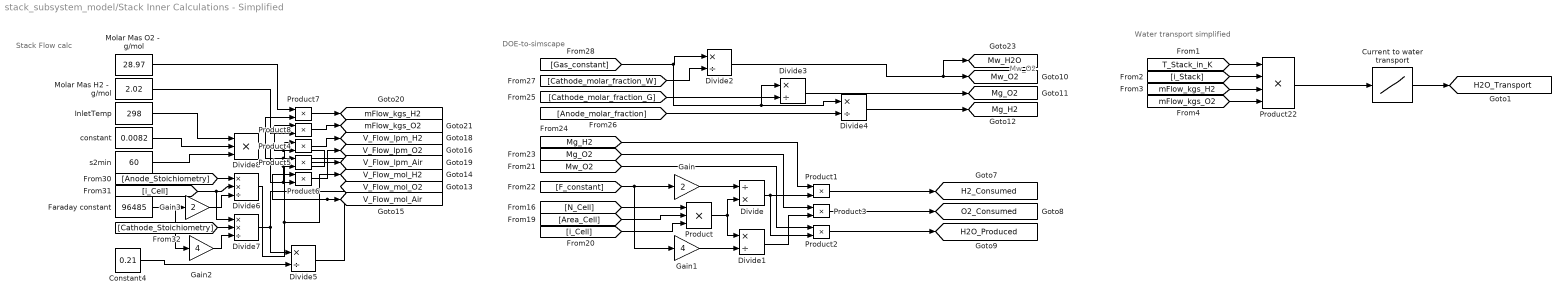
== system stack_subsystem_model/Stack Inner Calculations - Simplified ==
  note: DOE-to-simscape
  note: Stack Flow calc
  note: Mw_O2
  note: Water transport simplified
  Constant4 : Constant  Value=0.21
  Current to water transport : Lookup_n-D  NumberOfTableDimensions=1  BreakpointsForDimension1=[0:50:400]  Table=[0, 9932, 21438, 33442,47123, 59491, 77033, 93585, 112042]  InternalRulePriority=Speed  RndMeth=Simplest
  Divide : Product  Inputs=/*
  Divide{1..5} (5 alike) : Product  Inputs=*/
  Divide6 : Product  Inputs=**/
  Divide7 : Product  Inputs=**/
  Divide8 : Product  Inputs=***
  Faraday constant : Constant  Value=96485
  Gain : Gain  Gain=2
  Gain1 : Gain  Gain=4
  Gain2 : Gain  Gain=4
  Gain3 : Gain  Gain=2
  InletTemp : Constant  Value=298
  Molar Mas H2 -  g/mol : Constant  Value=2.02
  "Molar Mas O2 -  g/mol " : Constant  Value=28.97
  Product : Product  Inputs=3
  Product{1..8} (8 alike) : Product
  Product22 : Product  Inputs=4
  constant : Constant  Value=0.0082
  s2min : Constant  Value=60
  tag scope: H2O_Produced=global, H2O_Transport=global, H2_Consumed=global, Mg_H2=global, Mg_O2=global, Mw_H2O=global, Mw_O2=global, O2_Consumed=global, V_Flow_lpm_Air=global, V_Flow_lpm_H2=global, V_Flow_lpm_O2=global, V_Flow_mol_Air=global, V_Flow_mol_H2=global, V_Flow_mol_O2=global, mFlow_kgs_H2=global, mFlow_kgs_O2=global
  wires:
  Divide1/1 -> Product3/2
  Divide/1 -> Product1/2, Product2/2
  [Mg_O2] -> Product3/1
  [Mw_O2] -> Product2/1
  [Mg_H2] -> Product1/1
  Product3/1 -> [O2_Consumed]
  Product6/1 -> [V_Flow_lpm_Air]
  "Molar Mas O2 -  g/mol "/1 -> Product7/1
  Product2/1 -> [H2O_Produced]
  Molar Mas H2 -  g/mol/1 -> Product8/2
  Product7/1 -> [mFlow_kgs_H2]
  Product5/1 -> [V_Flow_lpm_O2]
  Product4/1 -> [V_Flow_lpm_H2]
  s2min/1 -> Divide8/3
  InletTemp/1 -> Divide8/1
  [Anode_Stoichiometry] -> Divide6/1
  Constant4/1 -> Divide5/2
  Gain2/1 -> Divide7/3
  Divide4/1 -> [Mg_H2]
  Divide3/1 -> [Mg_O2]
  Divide5/1 -> [V_Flow_mol_Air], Product6/1
  Divide2/1 -> [Mw_O2], [Mw_H2O]
  [Cathode_molar_fraction_G] -> Divide3/2
  [Anode_molar_fraction] -> Divide4/2
  [F_constant] -> Gain/1, Gain1/1
  Gain1/1 -> Divide1/2
  [i_Cell] -> Product/3
  Gain/1 -> Divide/1
  [i_Cell] -> Divide7/1, Divide6/2
  Faraday constant/1 -> Gain2/1, Gain3/1
  Gain3/1 -> Divide6/3
  Divide7/1 -> Divide5/1, Product5/1, Product7/2, [V_Flow_mol_O2]
  Product1/1 -> [H2_Consumed]
  Divide8/1 -> Product6/2, Product5/2, Product4/2, Product8/1
  [Cathode_Stoichiometry] -> Divide7/2
  constant/1 -> Divide8/2
  [N_Cell] -> Product/1
  [Gas_constant] -> Divide2/1, Divide4/1, Divide3/1
  Product8/1 -> [mFlow_kgs_O2]
  Divide6/1 -> Product4/1, [V_Flow_mol_H2]
  [Area_Cell] -> Product/2
  Product/1 -> Divide1/1, Divide/2
  [Cathode_molar_fraction_W] -> Divide2/2
  [mFlow_kgs_H2] -> Product22/3
  Current to water transport/1 -> [H2O_Transport]
  [i_Stack] -> Product22/2
  [T_Stack_in_K] -> Product22/1
  Product22/1 -> Current to water transport/1
  [mFlow_kgs_O2] -> Product22/4
